simulink model "SOC_Estimation_UKF"  (R2025b)
settings: Solver=VariableStepAuto  StartTime=0.0  StopTime=3200  RelTol=1e-3
model workspace (MAT data in the model file):
  Q = [1e-07  0  0; 0  1e-08  0; 0  0  1e-08]
  R = 0.5
  R1 = 0.35
  Tc = -0.1
  alpha = 0.7
  beta = 2
  k = 0
  n = 3
libraries: BatteryEstimators x1, dspfactors x1
(part 1 of 8)
settings Model: Creator=HP  LastModifiedBy=HP

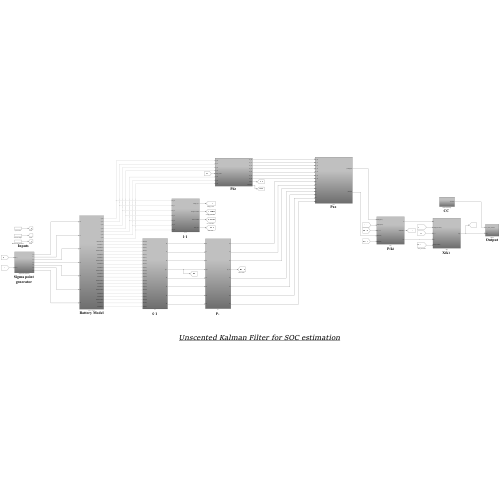
[thumbnail: Simulink's stored preview of the top-level diagram]
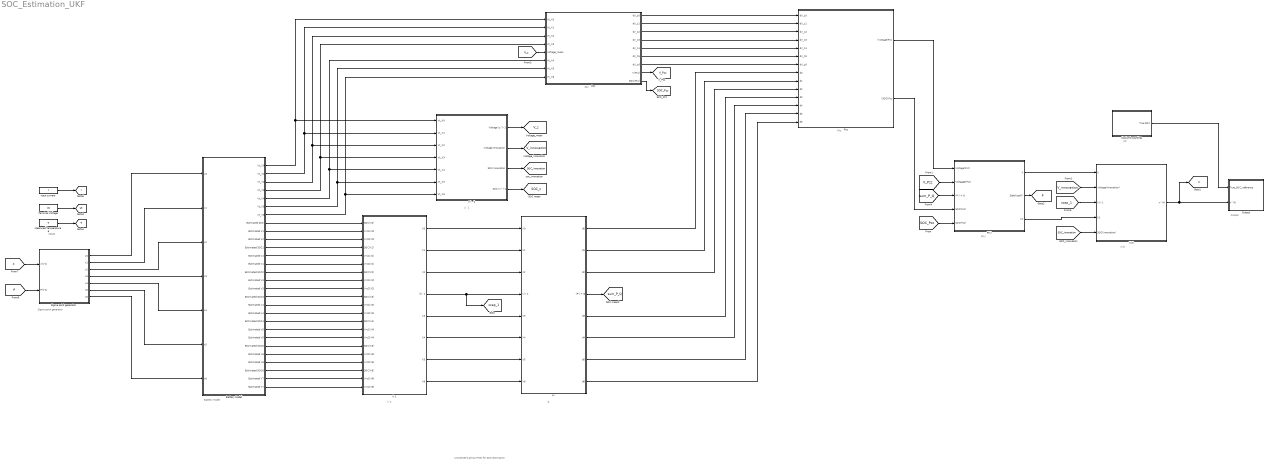
== system SOC_Estimation_UKF ==
  note: Inputs
  note: Sigma point generator
  note: Battery Model
  note: x̂⁻1
  note: P-
  note: ẑ ⁻1
  note: Pzz
  note: Pxz
  note: P(k)
  note: X(k)
  note: Output
  note: CC
  note: Unscented Kalman Filter for SOC estimation
  Battery Model : Subsystem
  "Coulumb counting " : Subsystem
  "Input current " : FromWorkspace  VariableName=I  SampleTime=0.1
  Measured Temperature 6 : FromWorkspace  VariableName=T  SampleTime=0.1
  Output : Subsystem
  P(k) : Subsystem
  P- : Subsystem
  Pxz : Subsystem
  Pzz : Subsystem
  "Sigma point generator " : Subsystem
  "Terminal Voltage " : FromWorkspace  VariableName=Vt  SampleTime=0.1
  X(k) : Subsystem
  x̂⁻1 : Subsystem
  z^−1 : Subsystem
  tag scope: I=global, P=global, SOC_Pzz=global, SOC_innovation=global, SOC_z=global, T=global, V_Pzz=global, V_innovation=global, V_z=global, Vt=global, X=global, sum_P_Q=global, xcap_1=global
  wires:
  Battery Model/5(Vt_X4) -> Pzz/6(Vt_X4), z^−1/5(Vt_X4)
  x̂⁻1/2(X1) -> P-/2(X1)
  x̂⁻1/8(X6) -> P-/8(X6)
  Battery Model/24(Estimated V6) -> x̂⁻1/17(Vrc1(X5))
  Battery Model/16(" Estimated V3") -> x̂⁻1/9(Vrc2(X2))
  Battery Model/12(Estimated V2) -> x̂⁻1/5(Vrc1(X1))
  x̂⁻1/5(X3) -> P-/5(X3)
  Battery Model/19(" Estimated V4") -> x̂⁻1/12(Vrc2(X3))
  Pzz/3(dV_z2) -> Pxz/3(dV_z2)
  Battery Model/2(Vt_X1) -> Pzz/2(Vt_X1), z^−1/2(Vt_X1)
  Battery Model/11(Estimated SOC1) -> x̂⁻1/4(SOC(X1))
  "Sigma point generator "/1(x0) -> Battery Model/1(x0)
  Battery Model/8(Estimated SOC) -> x̂⁻1/1(SOC(X0))
  Battery Model/20(Estimated SOC4) -> x̂⁻1/13(SOC(X4))
  "Sigma point generator "/2(x1) -> Battery Model/2(x1)
  P-/7(d5) -> Pxz/13(d5)
  x̂⁻1/7(X5) -> P-/7(X5)
  Battery Model/17(Estimated SOC3) -> x̂⁻1/10(SOC(X3))
  Battery Model/6(Vt_X5) -> Pzz/7(Vt_X5), z^−1/6(Vt_X5)
  Battery Model/3(Vt_X2) -> Pzz/3(Vt_X2), z^−1/3(Vt_X2)
  "Sigma point generator "/5(x4) -> Battery Model/5(x4)
  Battery Model/21(Estimated V5) -> x̂⁻1/14(Vrc1(X4))
  Battery Model/13(" Estimated V1") -> x̂⁻1/6(Vrc2(X1))
  Battery Model/15(Estimated V3) -> x̂⁻1/8(Vrc1(X2))
  Pzz/7(dV_z6) -> Pxz/7(dV_z6)
  P-/2(d1) -> Pxz/9(d1)
  P-/6(d4) -> Pxz/12(d4)
  Battery Model/4(Vt_X3) -> Pzz/4(Vt_X3), z^−1/4(Vt_X3)
  "Sigma point generator "/6(x5) -> Battery Model/6(x5)
  P(k)/1(K) -> X(k)/1(K)
  Battery Model/10(" Estimated V2") -> x̂⁻1/3(Vrc2(X0))
  Pxz/1((Voltage)Pxz) -> P(k)/1(Voltage(Pxz))
  x̂⁻1/3(X2) -> P-/3(X2)
  Battery Model/9(Estimated V1) -> x̂⁻1/2(Vrc1(X0))
  Pzz/2(dV_z1) -> Pxz/2(dV_z1)
  P-/1(d0) -> Pxz/8(d0)
  Battery Model/1(Vt_X0) -> Pzz/1(Vt_X0), z^−1/1(Vt_X0)
  "Sigma point generator "/4(x3) -> Battery Model/4(x3)
  Battery Model/27(Estimated V7) -> x̂⁻1/20(Vrc1(X6))
  P-/5(d3) -> Pxz/11(d3)
  Battery Model/22(" Estimated V5") -> x̂⁻1/15(Vrc2(X4))
  Pzz/1(dV_z0) -> Pxz/1(dV_z0)
  Battery Model/28(" Estimated V7") -> x̂⁻1/21(Vrc2(X6))
  "Sigma point generator "/7(x6) -> Battery Model/7(x6)
  x̂⁻1/6(X4) -> P-/6(X4)
  Battery Model/18(Estimated V4) -> x̂⁻1/11(Vrc1(X3))
  x̂⁻1/1(X0) -> P-/1(X0)
  "Sigma point generator "/3(x2) -> Battery Model/3(x2)
  Battery Model/14(Estimated SOC2) -> x̂⁻1/7(SOC(X2))
  Pzz/6(dV_z5) -> Pxz/6(dV_z5)
  Battery Model/7(Vt_X6) -> Pzz/8(Vt_X6), z^−1/7(Vt_X6)
  X(k)/1(x^(k)) -> [X], Output/2(x^(k))
  P-/8(d6) -> Pxz/14(d6)
  x̂⁻1/4((x̂)⁻1) -> P-/4((x̂)⁻1), [xcap_1]
  Pzz/5(dV_z4) -> Pxz/5(dV_z4)
  Battery Model/23(Estimated SOC5) -> x̂⁻1/16(SOC(X5))
  Battery Model/26(Estimated SOC6) -> x̂⁻1/19(SOC(X6))
  Pzz/4(dV_z3) -> Pxz/4(dV_z3)
  Battery Model/25(" Estimated V6") -> x̂⁻1/18(Vrc2(X5))
  P-/3(d2) -> Pxz/10(d2)
  z^−1/4(SOC (z^)-1) -> [SOC_z]
  z^−1/3(SOC Innovation) -> [SOC_innovation]
  Pxz/2((SOC)Pxz) -> P(k)/4(SOC(Pxz))
  P(k)/3(K1) -> X(k)/4(K1)
  [SOC_innovation] -> X(k)/5(SOC(Innovation))
  Pzz/9(SOC(Pzz)) -> [SOC_Pzz]
  [SOC_Pzz] -> P(k)/5(SOC(Pzz))
  Pzz/8(V(Pzz)) -> [V_Pzz]
  [V_Pzz] -> P(k)/2(Voltgage(Pzz))
  z^−1/2(Voltage Innovation) -> [V_innovation]
  [V_innovation] -> X(k)/2(Voltage(Innovation))
  z^−1/1(Voltage (z^)-1) -> [V_z]
  [V_z] -> Pzz/5(Voltage_mean)
  P-/4((P-) + Q) -> [sum_P_Q]
  [sum_P_Q] -> P(k)/3((P-) + Q)
  [xcap_1] -> X(k)/3((x̂)⁻1)
  "Coulumb counting "/1(True SOC) -> Output/1(True_SOC_reference)
  P(k)/2(Stabilized P) -> [P]
  [P] -> "Sigma point generator "/2(P(k-1))
  [X] -> "Sigma point generator "/1(x(k-1))
  Measured Temperature 6/1 -> [T]
  "Terminal Voltage "/1 -> [Vt]
  "Input current "/1 -> [I]

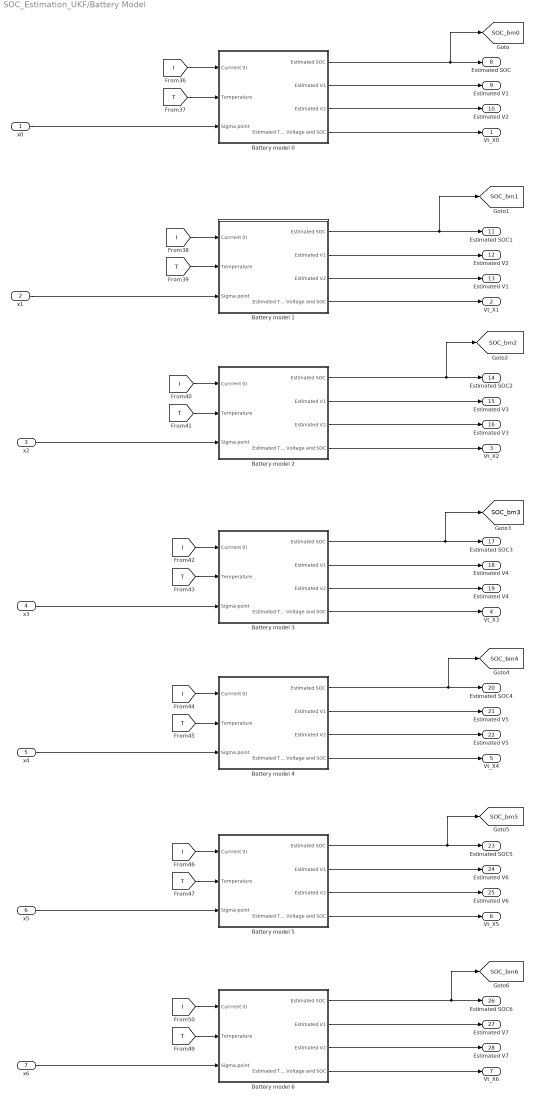
== system SOC_Estimation_UKF/Battery Model ==
  x0 : Inport
  x1 : Inport  Port=2
  x2 : Inport  Port=3
  x3 : Inport  Port=4
  x4 : Inport  Port=5
  x5 : Inport  Port=6
  x6 : Inport  Port=7
  Battery model 0 : Subsystem
  Battery model 1 : Subsystem
  Battery model 2 : Subsystem
  Battery model 3 : Subsystem
  Battery model 4 : Subsystem
  Battery model 5 : Subsystem
  Battery model 6 : Subsystem
  Vt_X0 : Outport
  Vt_X1 : Outport  Port=2
  Vt_X2 : Outport  Port=3
  Vt_X3 : Outport  Port=4
  Vt_X4 : Outport  Port=5
  Vt_X5 : Outport  Port=6
  Vt_X6 : Outport  Port=7
  Estimated SOC : Outport  Port=8
  Estimated V1 : Outport  Port=9
  " Estimated V2" : Outport  Port=10
  Estimated SOC1 : Outport  Port=11
  Estimated V2 : Outport  Port=12
  " Estimated V1" : Outport  Port=13
  Estimated SOC2 : Outport  Port=14
  Estimated V3 : Outport  Port=15
  " Estimated V3" : Outport  Port=16
  Estimated SOC3 : Outport  Port=17
  Estimated V4 : Outport  Port=18
  " Estimated V4" : Outport  Port=19
  Estimated SOC4 : Outport  Port=20
  Estimated V5 : Outport  Port=21
  " Estimated V5" : Outport  Port=22
  Estimated SOC5 : Outport  Port=23
  Estimated V6 : Outport  Port=24
  " Estimated V6" : Outport  Port=25
  Estimated SOC6 : Outport  Port=26
  Estimated V7 : Outport  Port=27
  " Estimated V7" : Outport  Port=28
  tag scope: SOC_bm0=global, SOC_bm1=global, SOC_bm2=global, SOC_bm3=global, SOC_bm4=global, SOC_bm5=global, SOC_bm6=global
  wires:
  Battery model 0/1(Estimated SOC) -> Estimated SOC/1, [SOC_bm0]
  [I] -> Battery model 2/1(Currrent (I))
  [I] -> Battery model 0/1(Currrent (I))
  Battery model 5/2(Estimated V1) -> Estimated V6/1
  Battery model 3/3(" Estimated V2") -> " Estimated V4"/1
  Battery model 2/2(Estimated V1) -> Estimated V3/1
  [T] -> Battery model 4/2("Temperature ")
  [I] -> Battery model 3/1(Currrent (I))
  [T] -> Battery model 2/2("Temperature ")
  x6/1 -> Battery model 6/3("Sigma point ")
  [I] -> Battery model 5/1(Currrent (I))
  [T] -> Battery model 3/2("Temperature ")
  [T] -> Battery model 6/2("Temperature ")
  [T] -> Battery model 0/2("Temperature ")
  Battery model 0/2(Estimated V1) -> Estimated V1/1
  [I] -> Battery model 1/1(Currrent (I))
  Battery model 1/1(Estimated SOC) -> Estimated SOC1/1, [SOC_bm1]
  [T] -> Battery model 1/2("Temperature ")
  Battery model 5/1(Estimated SOC) -> Estimated SOC5/1, [SOC_bm5]
  [I] -> Battery model 4/1(Currrent (I))
  Battery model 0/3(" Estimated V2") -> " Estimated V2"/1
  [I] -> Battery model 6/1(Currrent (I))
  Battery model 4/4(" Estimated Terminal Voltage and SOC") -> Vt_X4/1
  Battery model 2/3(" Estimated V2") -> " Estimated V3"/1
  Battery model 4/3(" Estimated V2") -> " Estimated V5"/1
  Battery model 1/2(Estimated V1) -> Estimated V2/1
  Battery model 0/4(" Estimated Terminal Voltage and SOC") -> Vt_X0/1
  [T] -> Battery model 5/2("Temperature ")
  Battery model 5/3(" Estimated V2") -> " Estimated V6"/1
  x5/1 -> Battery model 5/3("Sigma point ")
  Battery model 3/1(Estimated SOC) -> Estimated SOC3/1, [SOC_bm3]
  Battery model 4/1(Estimated SOC) -> Estimated SOC4/1, [SOC_bm4]
  x2/1 -> Battery model 2/3("Sigma point ")
  Battery model 4/2(Estimated V1) -> Estimated V5/1
  Battery model 6/3(" Estimated V2") -> " Estimated V7"/1
  Battery model 6/2(Estimated V1) -> Estimated V7/1
  x1/1 -> Battery model 1/3("Sigma point ")
  x4/1 -> Battery model 4/3("Sigma point ")
  Battery model 1/3(" Estimated V2") -> " Estimated V1"/1
  Battery model 3/2(Estimated V1) -> Estimated V4/1
  Battery model 2/1(Estimated SOC) -> Estimated SOC2/1, [SOC_bm2]
  Battery model 6/4(" Estimated Terminal Voltage and SOC") -> Vt_X6/1
  x0/1 -> Battery model 0/3("Sigma point ")
  Battery model 1/4(" Estimated Terminal Voltage and SOC") -> Vt_X1/1
  x3/1 -> Battery model 3/3("Sigma point ")
  Battery model 5/4(" Estimated Terminal Voltage and SOC") -> Vt_X5/1
  Battery model 2/4(" Estimated Terminal Voltage and SOC") -> Vt_X2/1
  Battery model 3/4(" Estimated Terminal Voltage and SOC") -> Vt_X3/1
  Battery model 6/1(Estimated SOC) -> [SOC_bm6], Estimated SOC6/1

== system SOC_Estimation_UKF/Coulumb counting  ==
  Constant1 : Constant
  SOC Estimator (Coulomb Counting) : BatteryEstimators/SOC Estimator (Coulomb Counting)  CurrentInputPartition=on  AH=2.9  Ts=0.1  DataType=Inherit: auto
      settings: LibrarySourceBlock=|
      | batt_sl_lib/Estimators/SOC Estimator
      | (Coulomb Counting)
  True SOC : Outport
  tag scope: SOC_cc=global
  wires:
  SOC Estimator (Coulomb Counting)/1 -> True SOC/1, [SOC_cc]  "Coulomb counting"
  Constant1/1 -> SOC Estimator (Coulomb Counting)/2
  [I] -> SOC Estimator (Coulomb Counting)/1

== system SOC_Estimation_UKF/Output ==
  note: UKF SOC estimate
  True_SOC_reference : Inport
  x^(k) : Inport  Port=2
  Demux : Demux  Outputs=3
  Real and estimated SOC : Scope  NumInputPorts=2
      settings: ActiveDisplayYMinimum=-0.055869733050867246  ActiveDisplayYMaximum=1.1173188592278742  DataLoggingVariableName=ScopeData8
  Subtract7 : Sum  Inputs=+-
  To Workspace : ToWorkspace  VariableName=error  SampleTime=-1
  wires:
  Subtract7/1 -> To Workspace/1
  True_SOC_reference/1 -> Real and estimated SOC/1, Subtract7/1
  Demux/1 -> Subtract7/2, Real and estimated SOC/2  "UKF SOC Estimate"
  x^(k)/1 -> Demux/1

== system SOC_Estimation_UKF/P(k) ==
  Voltage(Pxz) : Inport
  Voltgage(Pzz) : Inport  Port=2
  (P-) + Q : Inport  Port=3
  SOC(Pxz) : Inport  Port=4
  SOC(Pzz) : Inport  Port=5
  (K) : Product  Inputs=*/
  (K)1 : Product  Inputs=*/
  (P + Pt)/2 : Gain  Gain=0.5
  (Stabilized P) : Sum
  Jitter : Constant  Value=1e-5*eye(3)
  KPzz​KT : Product  Multiplication=Matrix(*)
  KPzz​KT1 : Product  Multiplication=Matrix(*)
  P : Sum  Inputs=+--
  P + Pt : Sum
  P transpose : Math  Operator=transpose
  Product1 : Product
  Product42 : Product
  Transpose1 : Math  Operator=transpose
  Transpose7 : Math  Operator=transpose
  K : Outport
  Stabilized P : Outport  Port=2
  K1 : Outport  Port=3
  wires:
  KPzz​KT/1 -> P/2
  (P-) + Q/1 -> P/1
  Product42/1 -> KPzz​KT/1
  (K)/1 -> K/1, Transpose7/1, Product42/1
  (P + Pt)/2/1 -> (Stabilized P)/1
  Transpose7/1 -> KPzz​KT/2
  P transpose/1 -> P + Pt/2
  P/1 -> P + Pt/1, P transpose/1
  Voltgage(Pzz)/1 -> (K)/2, Product42/2
  P + Pt/1 -> (P + Pt)/2/1
  Jitter/1 -> (Stabilized P)/2
  Voltage(Pxz)/1 -> (K)/1
  (Stabilized P)/1 -> Stabilized P/1
  SOC(Pxz)/1 -> (K)1/1
  SOC(Pzz)/1 -> Product1/2, (K)1/2
  (K)1/1 -> K1/1, Transpose1/1, Product1/1
  Product1/1 -> KPzz​KT1/1
  Transpose1/1 -> KPzz​KT1/2
  KPzz​KT1/1 -> P/3

== system SOC_Estimation_UKF/P- ==
  X0 : Inport
  X1 : Inport  Port=2
  X2 : Inport  Port=3
  (x̂)⁻1 : Inport  Port=4
  X3 : Inport  Port=5
  X4 : Inport  Port=6
  X5 : Inport  Port=7
  X6 : Inport  Port=8
  (P- + Q) : Sum
  (d0)​ : Sum  Inputs=+-
  (d1) : Sum  Inputs=+-
  (d2) : Sum  Inputs=+-
  (d3) : Sum  Inputs=+-
  (d4) : Sum  Inputs=+-
  (d5) : Sum  Inputs=+-
  (d6) : Sum  Inputs=+-
  M{0..6} (7 alike) : Product  Multiplication=Matrix(*)
  Product{7..13} (7 alike) : Product
  P− : Sum  Inputs=+++++++
  Q : Constant  Value=Q
  Transpose{,1..6} (7 alike) : Math  Operator=transpose
  d0 : Outport
  d1 : Outport  Port=2
  d2 : Outport  Port=3
  (P-) + Q : Outport  Port=4
  d3 : Outport  Port=5
  d4 : Outport  Port=6
  d5 : Outport  Port=7
  d6 : Outport  Port=8
  wires:
  Product12/1 -> P−/6
  M6/1 -> Product13/2
  M4/1 -> Product11/2
  M2/1 -> Product9/2
  Transpose2/1 -> M2/2
  M0/1 -> Product7/2
  (d4)/1 -> d4/1, M4/1, Transpose4/1
  Transpose5/1 -> M5/2
  (d0)​/1 -> d0/1, M0/1, Transpose/1
  X6/1 -> (d6)/1
  Product9/1 -> P−/3
  (d2)/1 -> d2/1, M2/1, Transpose2/1
  X0/1 -> (d0)​/1
  [wic] -> Product11/1
  Transpose6/1 -> M6/2
  (d5)/1 -> d5/1, Transpose5/1, M5/1
  Transpose4/1 -> M4/2
  (d1)/1 -> d1/1, M1/1, Transpose1/1
  (x̂)⁻1/1 -> (d5)/2, (d6)/2, (d4)/2, (d3)/2, (d2)/2, (d1)/2, (d0)​/2
  [wic] -> Product12/1
  [wic] -> Product13/1
  [wic] -> Product10/1
  Transpose/1 -> M0/2
  (d3)/1 -> d3/1, M3/1, Transpose3/1
  (P- + Q)/1 -> (P-) + Q/1
  Product7/1 -> P−/1
  Transpose1/1 -> M1/2
  (d6)/1 -> d6/1, Transpose6/1, M6/1
  M3/1 -> Product10/2
  X3/1 -> (d3)/1
  [w0c] -> Product7/1
  M5/1 -> Product12/2
  Q/1 -> (P- + Q)/2
  Product10/1 -> P−/4
  P−/1 -> (P- + Q)/1
  Product11/1 -> P−/5
  M1/1 -> Product8/2
  Transpose3/1 -> M3/2
  [wic] -> Product9/1
  Product13/1 -> P−/7
  Product8/1 -> P−/2
  X2/1 -> (d2)/1
  [wic] -> Product8/1
  X4/1 -> (d4)/1
  X5/1 -> (d5)/1
  X1/1 -> (d1)/1

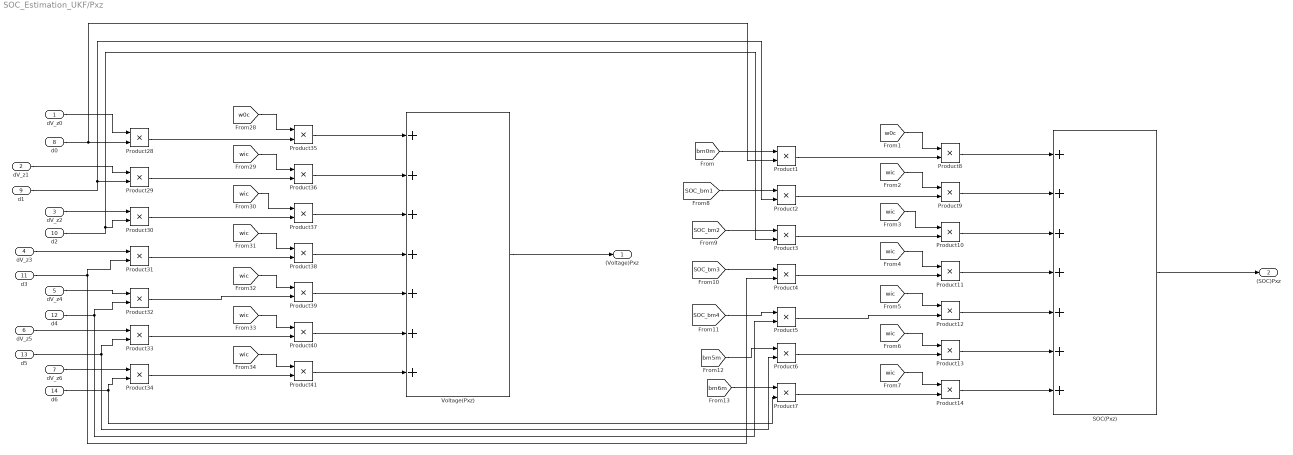
== system SOC_Estimation_UKF/Pxz ==
  dV_z0 : Inport
  dV_z1 : Inport  Port=2
  dV_z2 : Inport  Port=3
  dV_z3 : Inport  Port=4
  dV_z4 : Inport  Port=5
  dV_z5 : Inport  Port=6
  dV_z6 : Inport  Port=7
  d0 : Inport  Port=8
  d1 : Inport  Port=9
  d2 : Inport  Port=10
  d3 : Inport  Port=11
  d4 : Inport  Port=12
  d5 : Inport  Port=13
  d6 : Inport  Port=14
  Product{1..14,28..41} (28 alike) : Product
  SOC(Pxz)​ : Sum  Inputs=+++++++
  Voltage(Pxz)​ : Sum  Inputs=+++++++
  (Voltage)Pxz : Outport
  (SOC)Pxz : Outport  Port=2
  wires:
  [wic] -> Product39/1
  [wic] -> Product41/1
  Product32/1 -> Product39/2
  dV_z2/1 -> Product30/1
  [wic] -> Product38/1
  d6/1 -> Product34/2, Product7/2
  Product33/1 -> Product40/2
  [wic] -> Product36/1
  dV_z6/1 -> Product34/1
  [w0c] -> Product35/1
  Product38/1 -> Voltage(Pxz)​/4
  Product34/1 -> Product41/2
  dV_z4/1 -> Product32/1
  Product30/1 -> Product37/2
  [wic] -> Product40/1
  Product40/1 -> Voltage(Pxz)​/6
  Product39/1 -> Voltage(Pxz)​/5
  [wic] -> Product37/1
  dV_z5/1 -> Product33/1
  d3/1 -> Product31/2, Product4/2
  Product41/1 -> Voltage(Pxz)​/7
  Product35/1 -> Voltage(Pxz)​/1
  Product37/1 -> Voltage(Pxz)​/3
  Product28/1 -> Product35/2
  d5/1 -> Product33/2, Product6/2
  d0/1 -> Product28/2, Product1/2
  Product29/1 -> Product36/2
  Product31/1 -> Product38/2
  d4/1 -> Product32/2, Product5/2
  Product36/1 -> Voltage(Pxz)​/2
  d2/1 -> Product3/2, Product30/2
  dV_z0/1 -> Product28/1
  dV_z3/1 -> Product31/1
  Voltage(Pxz)​/1 -> (Voltage)Pxz/1
  dV_z1/1 -> Product29/1
  d1/1 -> Product29/2, Product2/2
  [wic] -> Product10/1
  Product9/1 -> SOC(Pxz)​/2
  Product8/1 -> SOC(Pxz)​/1
  [wic] -> Product11/1
  Product3/1 -> Product10/2
  Product1/1 -> Product8/2
  Product7/1 -> Product14/2
  [wic] -> Product13/1
  Product14/1 -> SOC(Pxz)​/7
  SOC(Pxz)​/1 -> (SOC)Pxz/1
  Product12/1 -> SOC(Pxz)​/5
  [wic] -> Product14/1
  [w0c] -> Product8/1
  [wic] -> Product9/1
  Product13/1 -> SOC(Pxz)​/6
  Product2/1 -> Product9/2
  Product11/1 -> SOC(Pxz)​/4
  Product5/1 -> Product12/2
  Product4/1 -> Product11/2
  Product10/1 -> SOC(Pxz)​/3
  Product6/1 -> Product13/2
  [wic] -> Product12/1
  [bm0m] -> Product1/1
  [SOC_bm1] -> Product2/1
  [SOC_bm2] -> Product3/1
  [SOC_bm3] -> Product4/1
  [SOC_bm4] -> Product5/1
  [bm5m] -> Product6/1
  [bm6m] -> Product7/1

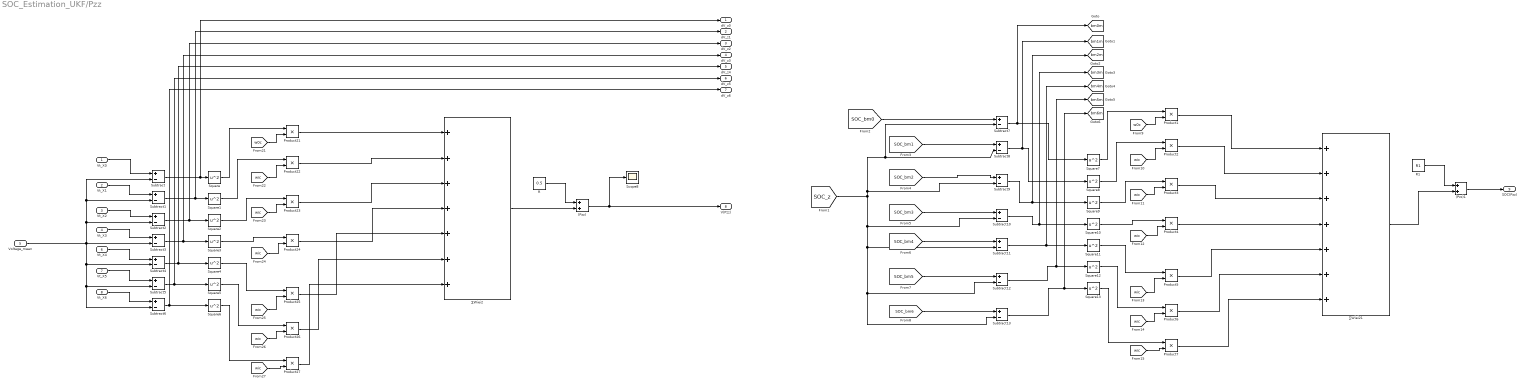
== system SOC_Estimation_UKF/Pzz ==
  Vt_X0 : Inport
  Vt_X1 : Inport  Port=2
  Vt_X2 : Inport  Port=3
  Vt_X3 : Inport  Port=4
  Voltage_mean : Inport  Port=5
  Vt_X4 : Inport  Port=6
  Vt_X5 : Inport  Port=7
  Vt_X6 : Inport  Port=8
  (Pzz) : Sum
  (Pzz)1 : Sum
  Product{1..7,21..27} (14 alike) : Product
  R : Constant  Value=0.5
  R1 : Constant  Value=R1
  Scope8 : Scope
      settings: ActiveDisplayYMinimum=9.9965634009257413E-6  ActiveDisplayYMaximum=1.0030938820403376E-5  DataLoggingVariableName=ScopeData2
  Square{,1..13} (14 alike) : Math  Operator=square
  Subtract{,1..13} (14 alike) : Sum  Inputs=+-
  ∑Wi​ei2​ : Sum  Inputs=+++++++
  ∑Wi​ei2​1 : Sum  Inputs=+++++++
  dV_z0 : Outport
  dV_z1 : Outport  Port=2
  dV_z2 : Outport  Port=3
  dV_z3 : Outport  Port=4
  dV_z4 : Outport  Port=5
  dV_z5 : Outport  Port=6
  dV_z6 : Outport  Port=7
  V(Pzz) : Outport  Port=8
  SOC(Pzz) : Outport  Port=9
  tag scope: bm0m=global, bm1m=global, bm2m=global, bm3m=global, bm4m=global, bm5m=global, bm6m=global
  wires:
  Subtract4/1 -> dV_z4/1, Square4/1
  Subtract2/1 -> dV_z2/1, Square2/1
  R/1 -> (Pzz)/1
  Subtract1/1 -> dV_z1/1, Square1/1
  Square3/1 -> Product24/1
  Subtract/1 -> dV_z0/1, Square/1
  Product24/1 -> ∑Wi​ei2​/4
  Product23/1 -> ∑Wi​ei2​/3
  [wic] -> Product24/2
  (Pzz)/1 -> V(Pzz)/1, Scope8/1
  [wic] -> Product22/2
  Subtract5/1 -> dV_z5/1, Square5/1
  Vt_X1/1 -> Subtract1/1
  [wic] -> Product25/2
  Square5/1 -> Product26/1
  Voltage_mean/1 -> Subtract1/2, Subtract/2, Subtract2/2, Subtract6/2, Subtract5/2, Subtract4/2, Subtract3/2
  Square6/1 -> Product27/1
  Square2/1 -> Product23/1
  Square1/1 -> Product22/1
  Subtract6/1 -> dV_z6/1, Square6/1
  [wic] -> Product23/2
  Vt_X3/1 -> Subtract3/1
  Product27/1 -> ∑Wi​ei2​/7
  Product21/1 -> ∑Wi​ei2​/1
  Subtract3/1 -> dV_z3/1, Square3/1
  Square/1 -> Product21/1
  Product25/1 -> ∑Wi​ei2​/5
  Square4/1 -> Product25/1
  ∑Wi​ei2​/1 -> (Pzz)/2
  [w0c] -> Product21/2
  Vt_X4/1 -> Subtract4/1
  Vt_X6/1 -> Subtract6/1
  Product26/1 -> ∑Wi​ei2​/6
  Vt_X0/1 -> Subtract/1
  [wic] -> Product27/2
  [wic] -> Product26/2
  Vt_X2/1 -> Subtract2/1
  Vt_X5/1 -> Subtract5/1
  Product22/1 -> ∑Wi​ei2​/2
  [SOC_bm6] -> Subtract13/1
  [SOC_bm1] -> Subtract8/1
  [SOC_bm3] -> Subtract10/1
  [SOC_bm4] -> Subtract11/1
  [SOC_bm5] -> Subtract12/1
  [SOC_bm2] -> Subtract9/1
  [SOC_bm0] -> Subtract7/1
  [SOC_z] -> Subtract10/2, Subtract13/2, Subtract12/2, Subtract11/2, Subtract9/2, Subtract7/2, Subtract8/2
  Square13/1 -> Product7/1
  [wic] -> Product4/2
  [wic] -> Product5/2
  [w0c] -> Product1/2
  Square7/1 -> Product1/1
  Square10/1 -> Product4/1
  [wic] -> Product2/2
  Product2/1 -> ∑Wi​ei2​1/2
  Product5/1 -> ∑Wi​ei2​1/5
  Product4/1 -> ∑Wi​ei2​1/4
  R1/1 -> (Pzz)1/1
  ∑Wi​ei2​1/1 -> (Pzz)1/2
  Product6/1 -> ∑Wi​ei2​1/6
  Product1/1 -> ∑Wi​ei2​1/1
  [wic] -> Product6/2
  [wic] -> Product7/2
  Product3/1 -> ∑Wi​ei2​1/3
  Square9/1 -> Product3/1
  Square11/1 -> Product5/1
  Product7/1 -> ∑Wi​ei2​1/7
  Square12/1 -> Product6/1
  Square8/1 -> Product2/1
  [wic] -> Product3/2
  Subtract7/1 -> Square7/1, [bm0m]
  Subtract8/1 -> [bm1m], Square8/1
  Subtract9/1 -> [bm2m], Square9/1
  Subtract10/1 -> [bm3m], Square10/1
  Subtract11/1 -> [bm4m], Square11/1
  Subtract12/1 -> [bm5m], Square12/1
  Subtract13/1 -> [bm6m], Square13/1
  (Pzz)1/1 -> SOC(Pzz)/1

== system SOC_Estimation_UKF/Sigma point generator  ==
  x(k-1) : Inport
  P(k-1) : Inport  Port=2
  Add : Sum
  Add1 : Sum
  Add2 : Sum
  Add3 : Sum  Inputs=+-
  Add4 : Sum  Inputs=+-
  Add5 : Sum  Inputs=+-
  "Cholesky Factor " : Subsystem
  S : Product
  S1 : Selector  NumberOfDimensions=2  InputPortWidth=3  IndexOptions=Select all,Index vector (dialog)  Indices=1,1  OutputSizes=1,1
  S2 : Selector  NumberOfDimensions=2  InputPortWidth=3  IndexOptions=Select all,Index vector (dialog)  Indices=1,2  OutputSizes=1,1
  S3 : Selector  NumberOfDimensions=2  InputPortWidth=3  IndexOptions=Select all,Index vector (dialog)  Indices=1,3  OutputSizes=1,1
  "UKF parameters " : Subsystem
  Unit Delay : UnitDelay  InitialCondition=[0.98;0;0]  SampleTime=-1  HasFrameUpgradeWarning=on
  Unit Delay1 : UnitDelay  InitialCondition=diag([0.05^2, 0.1^2, 0.1^2]);  SampleTime=-1  HasFrameUpgradeWarning=on
  x0 : Outport
  x1 : Outport  Port=2
  x2 : Outport  Port=3
  x3 : Outport  Port=4
  x4 : Outport  Port=5
  x5 : Outport  Port=6
  x6 : Outport  Port=7
  tag scope: w0c=global, w0m=global, wic=global, wim=global
  wires:
  "UKF parameters "/1(γ) -> S/2
  "Cholesky Factor "/1(L) -> S/1
  S/1 -> S3/1, S2/1, S1/1
  x(k-1)/1 -> Unit Delay/1
  S1/1 -> Add/2, Add4/2
  Add/1 -> x1/1
  S2/1 -> Add3/2, Add1/2
  Add1/1 -> x2/1
  S3/1 -> Add5/2, Add2/2
  Add2/1 -> x3/1
  Add4/1 -> x4/1
  Add3/1 -> x5/1
  Add5/1 -> x6/1
  P(k-1)/1 -> Unit Delay1/1
  "UKF parameters "/2(w0(m)) -> [w0m]
  "UKF parameters "/3(w1(m)) -> [wim]
  "UKF parameters "/4(w0(c)) -> [w0c]
  "UKF parameters "/5(w1(c)) -> [wic]
  Unit Delay/1 -> Add2/1, Add1/1, Add/1, Add5/1, Add3/1, Add4/1, x0/1
  Unit Delay1/1 -> "Cholesky Factor "/1(P)

== system SOC_Estimation_UKF/X(k) ==
  K : Inport
  Voltage(Innovation) : Inport  Port=2
  (x̂)⁻1 : Inport  Port=3
  K1 : Inport  Port=4
  SOC(Innovation) : Inport  Port=5
  (x^(k)) : Sum  Inputs=+++
  K(k)soc(k) : Product
  K(k)ν(k) : Product
  Kalman Demux : Demux  Outputs=3
  Kalman Demux1 : Demux  Outputs=3
  Scope : Scope
      settings: ActiveDisplayYMinimum=0.024617719792689913  ActiveDisplayYMaximum=0.042089569074477924  DataLoggingVariableName=ScopeData2  DataLoggingSaveFormat=Array
  Scope1 : Scope  NumInputPorts=3
      settings: ActiveDisplayYMinimum=-0.074758129634262538  ActiveDisplayYMaximum=0.091647323658433269
  Scope3 : Scope  NumInputPorts=3
      settings: ActiveDisplayYMinimum=-0.01848385022591071  ActiveDisplayYMaximum=0.034818923227962047  DataLoggingVariableName=ScopeData6
  x^(k) : Outport
  wires:
  K/1 -> K(k)ν(k)/2, Kalman Demux/1
  K(k)ν(k)/1 -> (x^(k))/1
  Kalman Demux/2 -> Scope3/2  "K(Vrc1)"
  (x̂)⁻1/1 -> (x^(k))/2
  Voltage(Innovation)/1 -> K(k)ν(k)/1
  Kalman Demux/3 -> Scope3/3  "K(Vrc2)"
  Kalman Demux/1 -> Scope3/1  "K(soc)"
  (x^(k))/1 -> x^(k)/1
  SOC(Innovation)/1 -> Scope/1, K(k)soc(k)/1
  K(k)soc(k)/1 -> (x^(k))/3
  K1/1 -> Kalman Demux1/1, K(k)soc(k)/2
  Kalman Demux1/3 -> Scope1/3  "K(Vrc2)"
  Kalman Demux1/2 -> Scope1/2  "K(Vrc1)"
  Kalman Demux1/1 -> Scope1/1  "K(soc)"

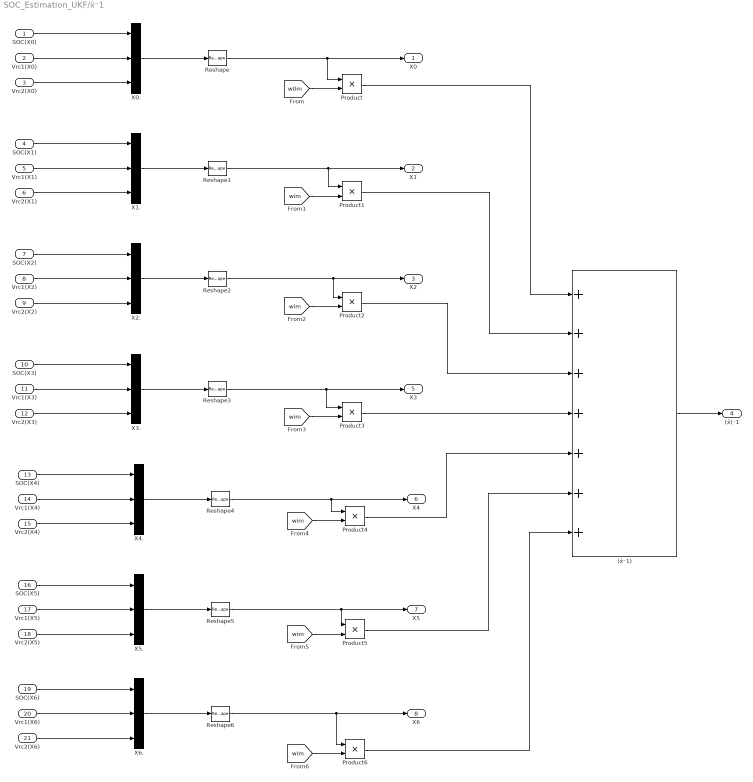
== system SOC_Estimation_UKF/x̂⁻1 ==
  SOC(X0) : Inport
  Vrc1(X0) : Inport  Port=2
  Vrc2(X0) : Inport  Port=3
  SOC(X1) : Inport  Port=4
  Vrc1(X1) : Inport  Port=5
  Vrc2(X1) : Inport  Port=6
  SOC(X2) : Inport  Port=7
  Vrc1(X2) : Inport  Port=8
  Vrc2(X2) : Inport  Port=9
  SOC(X3) : Inport  Port=10
  Vrc1(X3) : Inport  Port=11
  Vrc2(X3) : Inport  Port=12
  SOC(X4) : Inport  Port=13
  Vrc1(X4) : Inport  Port=14
  Vrc2(X4) : Inport  Port=15
  SOC(X5) : Inport  Port=16
  Vrc1(X5) : Inport  Port=17
  Vrc2(X5) : Inport  Port=18
  SOC(X6) : Inport  Port=19
  Vrc1(X6) : Inport  Port=20
  Vrc2(X6) : Inport  Port=21
  (x̂⁻1) : Sum  Inputs=+++++++
  Product{,1..6} (7 alike) : Product
  Reshape{,1..6} (7 alike) : Reshape  OutputDimensionality=Customize  OutputDimensions=[3,1]
  X0. : Mux  Inputs=3
  X1. : Mux  Inputs=3
  X2. : Mux  Inputs=3
  X3. : Mux  Inputs=3
  X4. : Mux  Inputs=3
  X5. : Mux  Inputs=3
  X6. : Mux  Inputs=3
  X0 : Outport
  X1 : Outport  Port=2
  X2 : Outport  Port=3
  (x̂)⁻1 : Outport  Port=4
  X3 : Outport  Port=5
  X4 : Outport  Port=6
  X5 : Outport  Port=7
  X6 : Outport  Port=8
  wires:
  Vrc2(X5)/1 -> X5./3
  Reshape/1 -> Product/1, X0/1
  SOC(X5)/1 -> X5./1
  [wim] -> Product6/2
  X3./1 -> Reshape3/1
  X0./1 -> Reshape/1
  Reshape6/1 -> X6/1, Product6/1
  [wim] -> Product2/2
  Vrc2(X4)/1 -> X4./3
  Product/1 -> (x̂⁻1)/1
  SOC(X2)/1 -> X2./1
  Reshape1/1 -> X1/1, Product1/1
  (x̂⁻1)/1 -> (x̂)⁻1/1
  Product5/1 -> (x̂⁻1)/6
  Product6/1 -> (x̂⁻1)/7
  Reshape2/1 -> X2/1, Product2/1
  Vrc2(X3)/1 -> X3./3
  X5./1 -> Reshape5/1
  Product2/1 -> (x̂⁻1)/3
  SOC(X3)/1 -> X3./1
  [wim] -> Product5/2
  [wim] -> Product3/2
  Vrc2(X0)/1 -> X0./3
  SOC(X0)/1 -> X0./1
  Reshape3/1 -> Product3/1, X3/1
  Vrc1(X3)/1 -> X3./2
  Reshape4/1 -> Product4/1, X4/1
  [wim] -> Product1/2
  [wim] -> Product4/2
  Product3/1 -> (x̂⁻1)/4
  Product1/1 -> (x̂⁻1)/2
  X4./1 -> Reshape4/1
  Vrc2(X1)/1 -> X1./3
  X1./1 -> Reshape1/1
  Reshape5/1 -> X5/1, Product5/1
  SOC(X6)/1 -> X6./1
  Vrc1(X4)/1 -> X4./2
  X6./1 -> Reshape6/1
  SOC(X4)/1 -> X4./1
  Vrc1(X0)/1 -> X0./2
  [w0m] -> Product/2
  Product4/1 -> (x̂⁻1)/5
  Vrc1(X1)/1 -> X1./2
  X2./1 -> Reshape2/1
  Vrc1(X6)/1 -> X6./2
  SOC(X1)/1 -> X1./1
  Vrc2(X6)/1 -> X6./3
  Vrc1(X2)/1 -> X2./2
  Vrc2(X2)/1 -> X2./3
  Vrc1(X5)/1 -> X5./2

== system SOC_Estimation_UKF/z^−1 ==
  Vt_X0 : Inport
  Vt_X1 : Inport  Port=2
  Vt_X2 : Inport  Port=3
  Vt_X3 : Inport  Port=4
  Vt_X4 : Inport  Port=5
  Vt_X5 : Inport  Port=6
  Vt_X6 : Inport  Port=7
  (Innovation2) : Sum  Inputs=+-
  Innovation : Sum  Inputs=+-
  Product{1..7,14..20} (14 alike) : Product
  SOC (z^−1) : Sum  Inputs=+++++++
  Scope4 : Scope
      settings: ActiveDisplayYMinimum=-0.049096174129987069  ActiveDisplayYMaximum=0.095599947621378856  DataLoggingVariableName=ScopeData7
  Scope6 : Scope  NumInputPorts=2
      settings: ActiveDisplayYMinimum=3.6027181272911375  ActiveDisplayYMaximum=4.2164807241409541  DataLoggingVariableName=ScopeData9
  To Workspace : ToWorkspace  VariableName=Verror  SampleTime=-1
  Voltage (z^−1) : Sum  Inputs=+++++++
  Voltage (z^)-1 : Outport
  Voltage Innovation : Outport  Port=2
  SOC Innovation : Outport  Port=3
  SOC (z^)-1 : Outport  Port=4
  wires:
  Product20/1 -> Voltage (z^−1)/1
  Product17/1 -> Voltage (z^−1)/6
  Product14/1 -> Voltage (z^−1)/3
  [wim] -> Product15/2
  Product15/1 -> Voltage (z^−1)/4
  Vt_X6/1 -> Product18/1
  Innovation/1 -> Voltage Innovation/1, To Workspace/1, Scope4/1
  [wim] -> Product17/2
  Product16/1 -> Voltage (z^−1)/5
  [wim] -> Product14/2
  [wim] -> Product19/2
  [w0m] -> Product20/2
  [wim] -> Product16/2
  Product18/1 -> Voltage (z^−1)/7
  Voltage (z^−1)/1 -> Voltage (z^)-1/1, Innovation/2, Scope6/2
  Vt_X2/1 -> Product14/1
  [Vt] -> Innovation/1, Scope6/1
  Product19/1 -> Voltage (z^−1)/2
  Vt_X0/1 -> Product20/1
  Vt_X4/1 -> Product16/1
  Vt_X1/1 -> Product19/1
  Vt_X5/1 -> Product17/1
  Vt_X3/1 -> Product15/1
  [wim] -> Product18/2
  Product3/1 -> SOC (z^−1)/5
  [SOC_bm4] -> Product3/1
  [SOC_cc] -> (Innovation2)/1
  [SOC_bm0] -> Product7/1
  [SOC_bm5] -> Product4/1
  [w0m] -> Product7/2
  Product5/1 -> SOC (z^−1)/7
  [wim] -> Product5/2
  [wim] -> Product1/2
  (Innovation2)/1 -> SOC Innovation/1
  Product4/1 -> SOC (z^−1)/6
  [wim] -> Product2/2
  Product1/1 -> SOC (z^−1)/3
  Product2/1 -> SOC (z^−1)/4
  [wim] -> Product4/2
  [wim] -> Product3/2
  [SOC_bm6] -> Product5/1
  SOC (z^−1)/1 -> (Innovation2)/2, SOC (z^)-1/1
  [wim] -> Product6/2
  [SOC_bm1] -> Product6/1
  [SOC_bm3] -> Product2/1
  Product7/1 -> SOC (z^−1)/1
  Product6/1 -> SOC (z^−1)/2
  [SOC_bm2] -> Product1/1
